simulink model "GPSIMUInputs"  (R2024b)
settings: configuration reference "STM32H7_Config" (kept outside this file)
settings Model: DataDictionary=Master_Dictionary.sldd  EnableAccessToBaseWorkspace=off  Creator=torni  LastModifiedBy=Will
settings ConfigSetRef: SourceName=STM32H7_Config

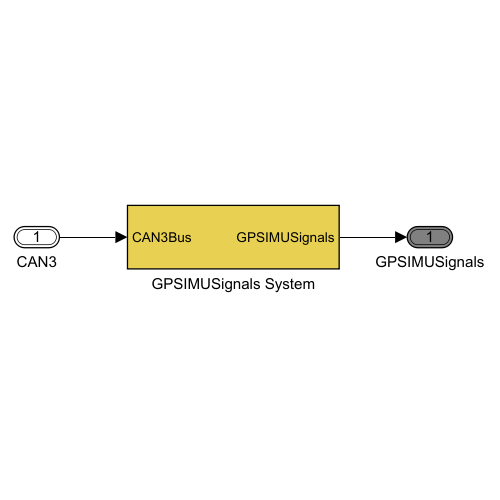
[thumbnail: Simulink's stored preview of the top-level diagram]
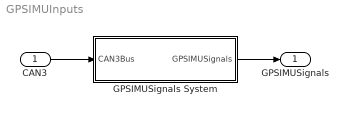
== system GPSIMUInputs ==
  CAN3 : Inport  OutDataTypeStr=Bus: CAN3Bus
  GPSIMUSignals System : Subsystem
  GPSIMUSignals : Outport  OutDataTypeStr=Bus: GPSIMUSignals  VectorParamsAs1DForOutWhenUnconnected=off
  wires:
  CAN3/1 -> GPSIMUSignals System/1(CAN3Bus)
  GPSIMUSignals System/1(GPSIMUSignals) -> GPSIMUSignals/1

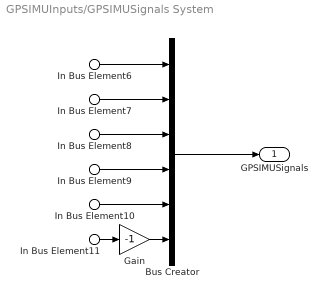
== system GPSIMUInputs/GPSIMUSignals System ==
  In Bus Element6 : Inport  PortName=CAN3Bus  Element=IMU.vLateralIMU
  In Bus Element7 : Inport  PortName=CAN3Bus  Element=IMU.gVerticalIMU
  In Bus Element8 : Inport  PortName=CAN3Bus  Element=IMU.vLongitudinalIMU
  In Bus Element9 : Inport  PortName=CAN3Bus  Element=IMU.gLateralIMU
  In Bus Element10 : Inport  PortName=CAN3Bus  Element=IMU.gLongitudinalIMU
  In Bus Element11 : Inport  PortName=CAN3Bus  Element=IMU.nYawRateIMU
  Bus Creator : BusCreator  Inputs=6  OutDataTypeStr=Bus: GPSIMUSignals
  Gain : Gain  Gain=-1
  GPSIMUSignals : Outport  OutDataTypeStr=Bus: GPSIMUSignals  VectorParamsAs1DForOutWhenUnconnected=off
  wires:
  Bus Creator/1 -> GPSIMUSignals/1
  In Bus Element6/1 -> Bus Creator/1
  In Bus Element7/1 -> Bus Creator/2
  In Bus Element8/1 -> Bus Creator/3
  In Bus Element9/1 -> Bus Creator/4
  In Bus Element10/1 -> Bus Creator/5
  In Bus Element11/1 -> Gain/1
  Gain/1 -> Bus Creator/6
